simulink model "hospital_scenario"  (R2023b)
settings: Solver=VariableStepAuto  StartTime=0.0  StopTime=10000.0  RelTol=1e-3
undefined symbols (not defined in the file or in its folder): control, entity, entitySys, get_finalDeparture, m
libraries: simulink x1
settings Model: Creator=francescafornasier  LastModifiedBy=valet
settings DebuggingCC: UnconnectedInputMsg=warning  UnconnectedOutputMsg=warning  UnconnectedLineMsg=warning
settings ModelReferenceCC: EnableRefExpFcnMdlSchedulingChecks=on
settings RTWCC: DLArmComputeVersion=19.05

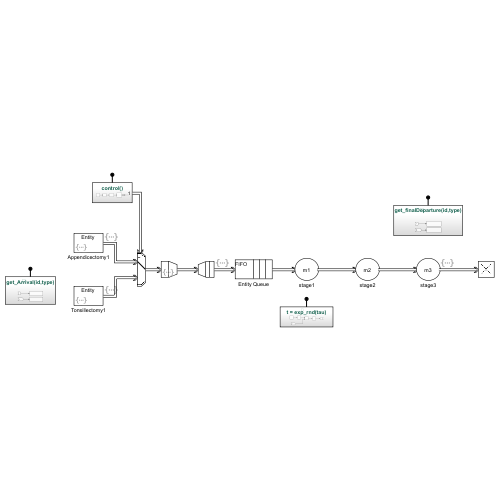
[thumbnail: Simulink's stored preview of the top-level diagram]
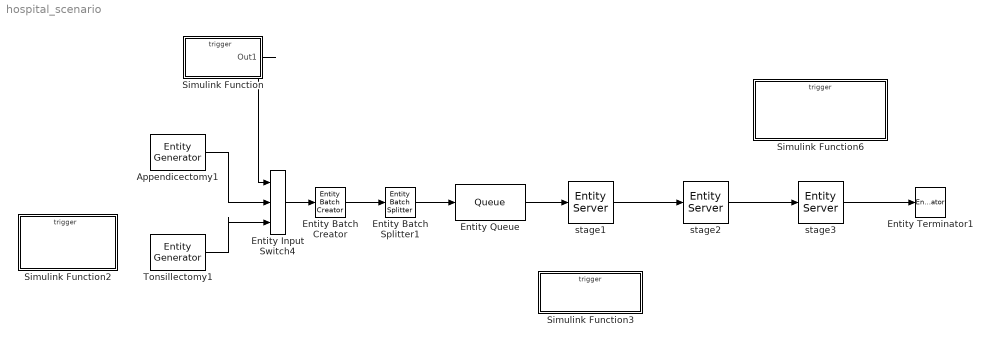
== system hospital_scenario ==
  Appendicectomy1 : EntityGenerator  OutputPortMessageModes=m  TimeSource=MATLAB action  IntergenerationTimeAction=|  GenerateEntityAtSimulationStart=off  GenerateAction=|  ExitAction=control()  AttributeName=type|tau_1|tau_2|tau_3  AttributeInitialValue=1|tau_A_1|tau_A_2|tau_A_3  EntityType=Structured  EntityTypeName=Entity
      IntergenerationTimeAction=|
      | persistent entityCounter_A igt_A;
      | if isempty(entityCounter_A)
      |     igt_A = [zeros(1,N/2) inf];
      |     entityCounter_A=1;
      | end
      | 
      | dt = igt_A(entityCounter_A);
      | entityCounter_A = entityCounter_A + 1; %Incrementa il contatore
      GenerateAction=|
      | entity.tau_1= exp_rnd(entity.tau_1);
      | entity.tau_2= exp_rnd(entity.tau_2);
      | entity.tau_3= exp_rnd(entity.tau_3);
  Entity Input Switch4 : EntityInputSwitch  InputPortMessageModes=m,m,m  OutputPortMessageModes=m  ActivePortSelection=Switch  SwitchingCriterion=From control port
      settings: InputPortMap=u0,u1,u2
  Entity Batch Creator : EntityBatchCreator  InputPortMessageModes=m  OutputPortMessageModes=m  NumberOfEntitiesInBatch=N  BatchGenerateAction=|
      | if opt == 1
      |     % Get the number of entities in the batch
      |     numEntities = length(entity.batch);
      | 
      |     % Initialize an array to store total service times
      |     serviceTimes = zeros(numEntities, 1);
      | 
      |     % Collect total service times for each entity
      |     for i = 1:numEntities
      |         serviceTimes(i) = entity.batch(i).tau_1 + entity.batch(i).tau_2 + entity.batch(i).tau_3;
      |     end
      | 
      |     % Initialize variables for the Greedy Heuristic
      |     sortedBatch = entity.batch;  % To store sorted entities
      |     selected = false(numEntities, 1);  % To track selected entities
      | 
      |     % Greedy selection process
      |     for j = 1:numEntities
      |         % Find the unselected entity with the shortest service time
      |         minServiceTime = inf;
      |         minIndex = -1;
      |         for k = 1:numEntities
      |             if ~selected(k) && serviceTimes(k) < minServiceTime
      |                 minServiceTime = serviceTimes(k);
      |                 minIndex = k;
      |             end
      |         end
      | 
      |         % Mark the selected entity and add it to the sorted batch
      |         selected(minIndex) = true;
      |         sortedBatch(j) = entity.batch(minIndex);  % Append to sorted batch
      |     end
      | 
      |     % Assign the sorted batch back to the entity batch
      |     entity.batch = sortedBatch;
      | end
      settings: OutputPortMap=o4
  Entity Batch Splitter1 : EntityBatchSplitter  InputPortMessageModes=m  OutputPortMessageModes=m
      settings: OutputPortMap=o4
  Entity Queue : Queue  InputPortMessageModes=m  OutputPortMessageModes=m  Capacity=inf  EntryAction=|
      | get_Arrival(entitySys.id, entity.type)
      | serviceTimes = entity.tau_1 + entity.tau_2 + entity.tau_3;
      | fprintf("Patient ID: %.0f OPERATION TYPE: %.0f SERVICE TIME %.2f\n", entitySys.id, entity.type, serviceTimes);
  Entity Terminator1 : EntityTerminator  InputPortMessageModes=m
  Simulink Function : Subsystem  TreatAsAtomicUnit=on
  Simulink Function2 : Subsystem  TreatAsAtomicUnit=on
  Simulink Function3 : Subsystem  TreatAsAtomicUnit=on
  Simulink Function6 : Subsystem  TreatAsAtomicUnit=on
  Tonsillectomy1 : EntityGenerator  OutputPortMessageModes=m  TimeSource=MATLAB action  IntergenerationTimeAction=|  GenerateEntityAtSimulationStart=off  GenerateAction=|  ExitAction=control()  AttributeName=type|tau_1|tau_2|tau_3  AttributeInitialValue=2|tau_T_1|tau_T_2|tau_T_3  EntityType=Structured  EntityTypeName=Entity
      IntergenerationTimeAction=|
      | persistent entityCounter_T igt_T;
      | if isempty(entityCounter_T)
      |     igt_T = [zeros(1,N/2) inf];
      |     entityCounter_T = 1;
      | end
      | 
      | dt = igt_T(entityCounter_T);
      | entityCounter_T = entityCounter_T + 1; %Incrementa il contatore
      GenerateAction=|
      | entity.tau_1= exp_rnd(entity.tau_1);
      | entity.tau_2= exp_rnd(entity.tau_2);
      | entity.tau_3= exp_rnd(entity.tau_3);
  stage1 : EntityServer  InputPortMessageModes=m  OutputPortMessageModes=m  Capacity=m1  ServiceTimeSource=Attribute  ServiceTimeAttributeName=entity.tau_1  ServiceTimeAction=dt = exp_rnd(entity.tau_1);
  stage2 : EntityServer  InputPortMessageModes=m  OutputPortMessageModes=m  Capacity=m2  ServiceTimeSource=Attribute  ServiceTimeAttributeName=entity.tau_2  ServiceTimeAction=dt = exp_rnd(entity.tau_2);
  stage3 : EntityServer  InputPortMessageModes=m  OutputPortMessageModes=m  Capacity=m3  ServiceTimeSource=Attribute  ServiceTimeAttributeName=entity.tau_3  ServiceTimeAction=dt = exp_rnd(entity.tau_3);  ExitAction=get_finalDeparture(entitySys.id, entity.type)
  wires:
  Entity Queue/1 -> stage1/1
  stage3/1 -> Entity Terminator1/1
  Tonsillectomy1/1 -> Entity Input Switch4/3
  Entity Batch Splitter1/1 -> Entity Queue/1
  stage1/1 -> stage2/1
  stage2/1 -> stage3/1
  Appendicectomy1/1 -> Entity Input Switch4/2
  Simulink Function/1(Out1) -> Entity Input Switch4/1
  Entity Batch Creator/1 -> Entity Batch Splitter1/1
  Entity Input Switch4/1 -> Entity Batch Creator/1

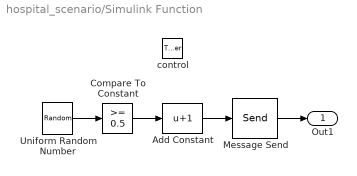
== system hospital_scenario/Simulink Function ==
  control : TriggerPort  TriggerType=function-call  IsSimulinkFunction=on  FunctionName=control  FunctionVisibility=scoped  VariantControl=(inherit)
  Add Constant : Bias  Bias=1  SaturateOnIntegerOverflow=off
  Compare To Constant : simulink/Logic and Bit Operations/Compare To Constant  relop=>=  const=0.5  OutDataTypeStr=uint8
  Message Send : Send  OutputPortMessageModes=m
  Uniform Random Number : UniformRandomNumber  Minimum=0  Seed=500
  Out1 : Outport
  wires:
  Uniform Random Number/1 -> Compare To Constant/1
  Message Send/1 -> Out1/1
  Compare To Constant/1 -> Add Constant/1
  Add Constant/1 -> Message Send/1

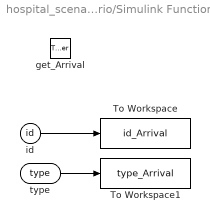
== system hospital_scenario/Simulink Function2 ==
  get_Arrival : TriggerPort  TriggerType=function-call  IsSimulinkFunction=on  FunctionName=get_Arrival  FunctionVisibility=scoped  VariantControl=(inherit)
  To Workspace : ToWorkspace  VariableName=id_Arrival  SaveFormat=Timeseries  SampleTime=-1
  To Workspace1 : ToWorkspace  VariableName=type_Arrival  SaveFormat=Timeseries  SampleTime=-1
  id : ArgIn  ArgumentName=id
  type : ArgIn  Port=2  ArgumentName=type
  wires:
  id/1 -> To Workspace/1
  type/1 -> To Workspace1/1

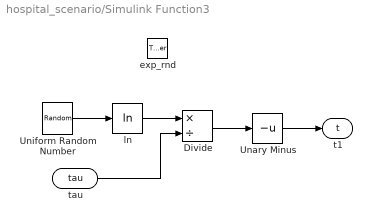
== system hospital_scenario/Simulink Function3 ==
  exp_rnd : TriggerPort  TriggerType=function-call  IsSimulinkFunction=on  FunctionName=exp_rnd  FunctionVisibility=scoped  VariantControl=(inherit)
  Divide : Product  Inputs=*/
  Unary Minus : UnaryMinus
  Uniform Random Number : UniformRandomNumber  Minimum=0
  ln : Math  Operator=log
  tau : ArgIn  ArgumentName=tau
  t1 : ArgOut  ArgumentName=t
  wires:
  Uniform Random Number/1 -> ln/1
  ln/1 -> Divide/1
  tau/1 -> Divide/2
  Divide/1 -> Unary Minus/1
  Unary Minus/1 -> t1/1

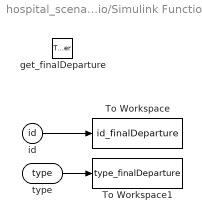
== system hospital_scenario/Simulink Function6 ==
  get_finalDeparture : TriggerPort  TriggerType=function-call  IsSimulinkFunction=on  FunctionName=get_finalDeparture  FunctionVisibility=scoped  VariantControl=(inherit)
  To Workspace : ToWorkspace  VariableName=id_finalDeparture  SaveFormat=Timeseries  SampleTime=-1
  To Workspace1 : ToWorkspace  VariableName=type_finalDeparture  SaveFormat=Timeseries  SampleTime=-1
  id : ArgIn  ArgumentName=id
  type : ArgIn  Port=2  ArgumentName=type
  wires:
  id/1 -> To Workspace/1
  type/1 -> To Workspace1/1
